simulink model "atrias_3d"  (R2014b)
settings: Solver=ode45  StartTime=0.0  StopTime=t_end  FixedStep=0.001  MaxStep=1e-2  RelTol=1e-3
InitFcn:
  | colors
  | simulation_params
  | mechanical_params
StartFcn:
  | tic
StopFcn:
  | stopscript
values from neighbouring files (symbols this model uses):
  b_hmotor = 0    [mechanical_params.m]
  b_leg_spring = 0.075*sqrt(k_leg_spring*0.5*.25^2)    [mechanical_params.m]
  b_rotor = 0*60/(2*pi)*9.725e-5    (= 0)    [mechanical_params.m]
  breakaway_friction = [25 25 25 25]    [mechanical_params.m]
  coulomb_friction = [20 20 20 20]    [mechanical_params.m]
  d_com = (d_hip_com_to_torso_com*m_torso)/(m_torso + num_legs*m_hshaft)    [mechanical_params.m]
  delta_phi_max = 160*pi/180    (= 2.79252680319)    [mechanical_params.m]
  delta_phi_min = 25.5*pi/180    (= 0.445058959259)    [mechanical_params.m]
  friction_linear_zone = [0.5 0.5 0.5 0.5].*pi/180    [mechanical_params.m]
  g = 9.81    [mechanical_params.m]
  HIP_MTR_MAX_TORQUE = max_current_hip*Kt_hip*N_h    (= 629.28)    [mechanical_params.m]
  initial_dx = -1    [mechanical_params.m]
  initial_hip_roll = 0    [mechanical_params.m]
  initial_pitch_joint_height = initial_com_height + boom_mount_to_com    [mechanical_params.m]
  initial_torso_pitch = 0*pi/180    (= 0)    [mechanical_params.m]
  initial_torso_roll = 0*pi/180    (= 0)    [mechanical_params.m]
  initial_torso_yaw = 0*pi/180    (= 0)    [mechanical_params.m]
  k_gx = m_total*g/0.01    (= 57082.15332)    [mechanical_params.m]
  k_gy = m_total*g/0.005    (= 114164.30664)    [mechanical_params.m]
  k_leg_spring = 2950    [mechanical_params.m]
  k_phi = 5000    [mechanical_params.m]
  Kb_leg = 0.121    [mechanical_params.m]
  Kt_leg = 0.121    [mechanical_params.m]
  L_leg = 0.102e-3    (= 0.000102)    [mechanical_params.m]
  l_seg = 0.5    [mechanical_params.m]
  LEG_MTR_MAX_TORQUE = max_current_leg * Kt_leg * N    (= 1210)    [mechanical_params.m]
  lowerleg_12 = 0.40    (= 0.4)    [mechanical_params.m]
  m_fblink = 0.46    [mechanical_params.m]
  m_hshaft = 18    [mechanical_params.m]
  m_lowerleg = 0.4438    [mechanical_params.m]
  m_output_gear = 1e-5    (= 1e-05)    [mechanical_params.m]
  m_rotor = 1e-5    (= 1e-05)    [mechanical_params.m]
  m_shin = 0.75    [mechanical_params.m]
  m_thigh = 0.69    [mechanical_params.m]
  m_torso = 17.5    [mechanical_params.m]
  m_total = num_legs*(m_hshaft + m_thigh + m_lowerleg + m_shin + m_fblink + 2*m_gearing) + m_torso    (= 58.18772)    [mechanical_params.m]
  m_virtual_gear = 1e-5    (= 1e-05)    [mechanical_params.m]
  max_current_leg = 200    [mechanical_params.m]
  max_voltage_leg = 50    [mechanical_params.m]
  mu_hmotor = 0.90    (= 0.9)    [mechanical_params.m]
  mu_motor = 0.85    [mechanical_params.m]
  mu_slide = 0.95    [mechanical_params.m]
  mu_stick = 1.00    (= 1)    [mechanical_params.m]
  N = 50    [mechanical_params.m]
  N_h = r_hip_shaft / r_hip_gearhead    (= 57)    [mechanical_params.m]
  phi_max_collision = -5*pi/180    (= -0.0872664625997)    [mechanical_params.m]
  phi_roll_max = pi + 16*pi/180    (= 3.42084533391)    [mechanical_params.m]
  phi_roll_min = pi - 9*pi/180    (= 2.98451302091)    [mechanical_params.m]
  phi_shin_max = 3*pi/2 + 17.5*pi/180    (= 5.01782159948)    [mechanical_params.m]
  phi_shin_min = pi - 45*pi/180    (= 2.35619449019)    [mechanical_params.m]
  phi_thigh_max = pi + 45*pi/180    (= 3.92699081699)    [mechanical_params.m]
  phi_thigh_min = pi/2 - 17.5*pi/180    (= 1.2653637077)    [mechanical_params.m]
  r_hip_gearhead = 0.009525    [mechanical_params.m]
  r_hip_shaft = 0.542925    [mechanical_params.m]
  R_leg = 0.052    [mechanical_params.m]
  r_rotor = 0.001    [mechanical_params.m]
  r_virtual_gear = N*r_rotor    (= 0.05)    [mechanical_params.m]
  shin_12 = 0.40    (= 0.4)    [mechanical_params.m]
  shin_initial_l = initial_l_leg_angle + acos(initial_l_leg_length)    [mechanical_params.m]
  shin_initial_r = initial_r_leg_angle + acos(initial_r_leg_length)    [mechanical_params.m]
  thigh_initial_l = initial_l_leg_angle - acos(initial_l_leg_length)    [mechanical_params.m]
  thigh_initial_r = initial_r_leg_angle - acos(initial_r_leg_length)    [mechanical_params.m]
  v_gx_max = 0.03    [mechanical_params.m]
  v_gy_max = 0.03    [mechanical_params.m]
  v_phi_max = 1/60    (= 0.0166666666667)    [mechanical_params.m]
  viscous_friction = [0.001 0.001 0.001 0.001]    [mechanical_params.m]
  vLimit = 0.01    [mechanical_params.m]
undefined symbols (not defined in the file or in its folder): A_lpf_velocity, B1_lpf_velocity, B2_lpf_velocity, fblink_color_d, floor_color_d, hshaft_color_d, lowerleg_color_d, output_sample_time, rad, s, sample_time, sgn, shin_color_d, t_friction, thigh_color_d, torso_color_d, X, Y, Z
libraries: sm_lib x163, nesl_utility x116, simulink x47, fl_lib x16, simulink_extras x2, mblibv1 x2, commnoisgen2 x1
(part 1 of 7)
settings Model: Creator=wmartin  LastModifiedBy=jonesmik
settings SolverCC: InitialStep=sample_time  MaxOrder=2  ConsecutiveZCsStepRelTol=auto  MaxConsecutiveZCs=auto  ZeroCrossControl=DisableAll  ZeroCrossAlgorithm=Adaptive  InsertRTBMode=Never (minimum delay)
settings DataIOCC: LimitDataPoints=off  SaveOutput=off  SignalLogging=off  DSMLogging=off  OutputOption=SpecifiedOutputTimes  OutputTimes=[0:output_sample_time:t_end]
settings OptimizationCC: InlineParams=on  UseDivisionForNetSlopeComputation=UseDivisionForReciprocalsOfIntegersOnly  UseFloatMulNetSlope=on  InlineInvariantSignals=on  EnhancedBackFolding=on  MemcpyThreshold=1024  StateBitsets=on  DataBitsets=on  EfficientFloat2IntCast=on  SimCompilerOptimization=On  AccelVerboseBuild=on
settings DebuggingCC: AlgebraicLoopMsg=none  UnderspecifiedInitializationDetection=Classic  MergeDetectMultiDrivingBlocksExec=none  SolverPrmCheckMsg=none  UnconnectedInputMsg=none  UnconnectedOutputMsg=none  UnconnectedLineMsg=none  StateNameClashWarn=warning
settings SFSimCC: SFSimEnableDebug=off  SFSimOverflowDetection=off  SFSimEcho=off
settings RTWCC: BuildConfiguration=Faster Runs
settings SimscapeCC: EditingMode=Restricted
settings ExplorerConfigSet: InternalSimMechanicsExplorerSettings="<ExplorerConfiguration><canonicalview>default</canonicalview><AnimationSetting><BasePlaybackSpeed>1.0</BasePlaybackSpeed><PlaybackSpeedFactor>1.0</PlaybackSpeedFactor></AnimationSetting><TilePanel><TileInfo><Tiles Columns=\"1\" Count=\"1\" Rows=\"1\"><Column Left=\"2\" Weight=\"1\"/><Column Left=\"876\"/><Row Top=\"2\" Weight=\"1\"/><Row Top=\"1114\"/><Tile Height=\"1\" Width=\"1\" X=\"0\" Y=\"0\"/></Tiles></TileInfo><SceneInfo><SceneViewer><BGColor><R>0.89803922176361084</R><G>0.89803922176361084</G><B>0.94901961088180542</B></BGColor><Camera><Position><X>-30.49227767907372</X><Y>0.073515473804125403</Y><Z>1.0865448159450428</Z></Position><Center><X>0</X><Y>0.073515473804125403</Y><Z>1.0865448159450428</Z></Center><Up><X>0</X><Y>0</Y><Z>1</Z></Up><Left>-3.5820650684649178</Left><Right>3.5820650684649178</Right><Bottom>-0.28042415136526933</Bottom><Top>0.28042415136526933</Top></Camera></SceneViewer></SceneInfo></TilePanel></ExplorerConfiguration>"

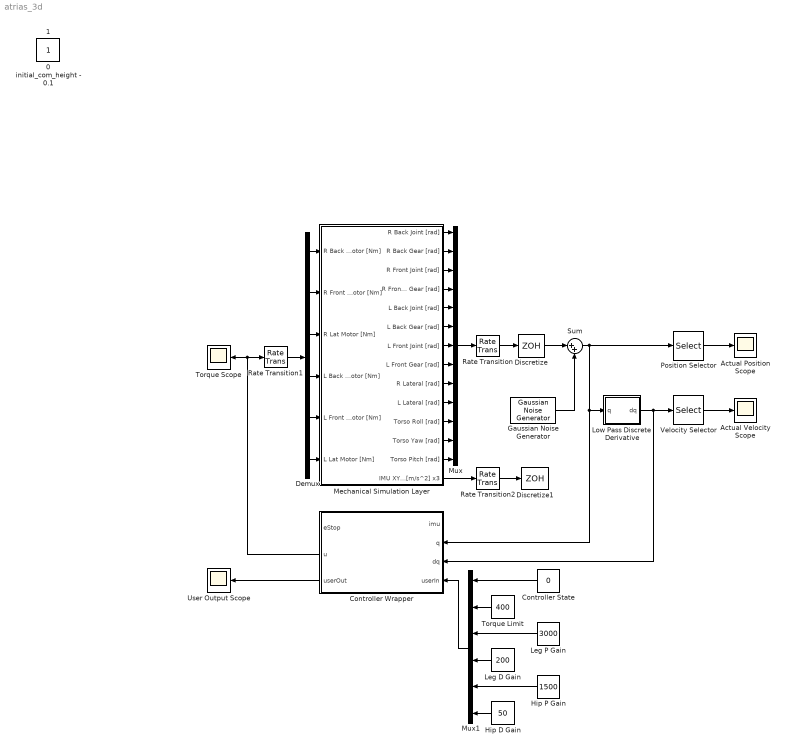
== system atrias_3d ==
  Actual Position Scope : Scope
      settings: SaveName=ScopeData7
  Actual Velocity Scope : Scope
      settings: YMin=-8  YMax=4  SaveName=ScopeData8
  Controller State : Constant  Value=0
  Controller Wrapper : MATLAB Function  TreatAsAtomicUnit=on
  Demux : Demux  Outputs=6
  Discretize : ZeroOrderHold  SampleTime=sample_time
  Discretize1 : ZeroOrderHold  SampleTime=sample_time
  Gaussian Noise Generator : commnoisgen2/Gaussian Noise Generator  m=0  d=sensor_noise_variance  s=41  Ts=sample_time  frameBased=off  sampPerFrame=1  orient=off  outDataType=double
  Hip D Gain : Constant  Value=50
  Hip P Gain : Constant  Value=1500
  Leg D Gain : Constant  Value=200
  Leg P Gain : Constant  Value=3000
  Low Pass Discrete Derivative : Subsystem
  Mechanical Simulation Layer : Subsystem
      mask Display: image('biped.jpg')
  Mux : Mux  Inputs=13
  Mux1 : Mux  Inputs=6
  Position Selector : Selector  InputPortWidth=13  IndexOptions=Select all  Indices=[13]
  Rate Transition : RateTransition  OutPortSampleTime=sample_time
  Rate Transition1 : RateTransition  OutPortSampleTime=sample_time
  Rate Transition2 : RateTransition  OutPortSampleTime=sample_time
  Sum : Sum  Inputs=|++
  Torque Scope : Scope
      settings: SaveName=ScopeData5
  Torque Limit : Constant  Value=400
  User Output Scope : Scope
      settings: YMin=0.12  YMax=0.28  SaveName=ScopeData4
  Velocity Selector : Selector  InputPortWidth=13  IndexOptions=Select all  Indices=[13]
  0 : Constant  IOType=siggen
  1 : Constant  IOType=siggen
  initial_com_height - 0.1 : Constant  IOType=siggen
  wires:
  Mechanical Simulation Layer/1(R Back Joint [rad]) -> Mux/1
  Mechanical Simulation Layer/2(R Back Gear [rad]) -> Mux/2
  Mechanical Simulation Layer/3(R Front Joint [rad]) -> Mux/3
  Mechanical Simulation Layer/4(R Front Gear [rad]) -> Mux/4
  Mechanical Simulation Layer/5(L Back Joint [rad]) -> Mux/5
  Mechanical Simulation Layer/6(L Back Gear [rad]) -> Mux/6
  Mechanical Simulation Layer/7(L Front Joint [rad]) -> Mux/7
  Mechanical Simulation Layer/8(L Front Gear [rad]) -> Mux/8
  Mechanical Simulation Layer/9(R Lateral [rad]) -> Mux/9
  Mechanical Simulation Layer/10(L Lateral [rad]) -> Mux/10
  Mechanical Simulation Layer/11(Torso Roll [rad]) -> Mux/11
  Mechanical Simulation Layer/12(Torso Yaw [rad]) -> Mux/12
  Mechanical Simulation Layer/13(Torso Pitch [rad]) -> Mux/13
  Demux/1 -> Mechanical Simulation Layer/1(R Back Motor [Nm])
  Demux/2 -> Mechanical Simulation Layer/2(R Front Motor [Nm])
  Demux/3 -> Mechanical Simulation Layer/3(R Lat Motor [Nm])
  Demux/4 -> Mechanical Simulation Layer/4(L Back Motor [Nm])
  Demux/5 -> Mechanical Simulation Layer/5(L Front Motor [Nm])
  Demux/6 -> Mechanical Simulation Layer/6(L Lat Motor [Nm])
  Rate Transition1/1 -> Demux/1
  Discretize/1 -> Sum/1
  Gaussian Noise Generator/1 -> Sum/2
  Rate Transition/1 -> Discretize/1
  Mux/1 -> Rate Transition/1
  Mechanical Simulation Layer/14("IMU XYZ Acclerations [m/s^2] x3 ") -> Rate Transition2/1
  Rate Transition2/1 -> Discretize1/1
  Sum/1 -> Position Selector/1, Controller Wrapper/2(q), Low Pass Discrete Derivative/1(q)
  Low Pass Discrete Derivative/1(dq) -> Velocity Selector/1, Controller Wrapper/3(dq)
  Controller Wrapper/2(u) -> Rate Transition1/1, Torque Scope/1
  Controller Wrapper/3(userOut) -> User Output Scope/1
  Mux1/1 -> Controller Wrapper/4(userIn)
  Controller State/1 -> Mux1/1
  Torque Limit/1 -> Mux1/2
  Leg P Gain/1 -> Mux1/3
  Leg D Gain/1 -> Mux1/4
  Hip P Gain/1 -> Mux1/5
  Hip D Gain/1 -> Mux1/6
  Position Selector/1 -> Actual Position Scope/1
  Velocity Selector/1 -> Actual Velocity Scope/1

== system atrias_3d/Low Pass Discrete Derivative ==
  q : Inport
  Gain1 : Gain  Gain=1/sample_time
  discrete difference : Subsystem
  two_pole_filter : DiscreteTransferFcn  Numerator=[A_lpf_velocity 0 0]  Denominator=[1 B1_lpf_velocity B2_lpf_velocity]  SampleTime=sample_time
  dq : Outport
  wires:
  discrete difference/1(out) -> Gain1/1
  Gain1/1 -> two_pole_filter/1
  two_pole_filter/1 -> dq/1
  q/1 -> discrete difference/1(in)

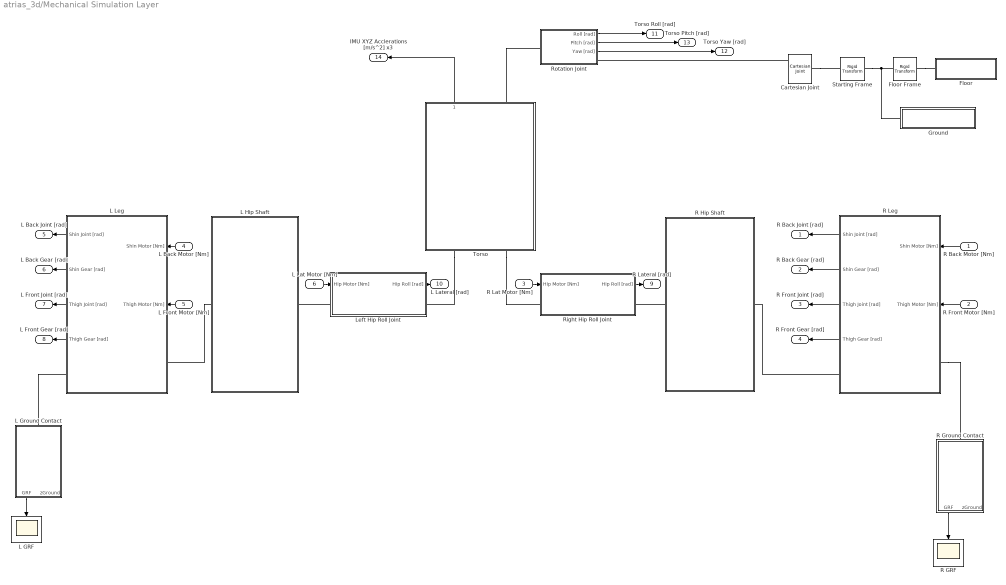
== system atrias_3d/Mechanical Simulation Layer ==
  R Back Motor [Nm] : Inport
  R Front Motor [Nm] : Inport  Port=2
  R Lat Motor [Nm] : Inport  Port=3
  L Back Motor [Nm] : Inport  Port=4
  L Front Motor [Nm] : Inport  Port=5
  L Lat Motor [Nm] : Inport  Port=6
  Cartesian Joint : sm_lib/Joints/Cartesian Joint  SenseConstraintForce=off  SenseConstraintForceX=off  SenseConstraintForceY=off  SenseConstraintForceZ=off  SenseConstraintTorque=off  SenseConstraintTorqueX=off  SenseConstraintTorqueY=off  SenseConstraintTorqueZ=off  SenseTotalForce=off  SenseTotalForceX=off  SenseTotalForceY=off  SenseTotalForceZ=off  SenseTotalTorque=off  SenseTotalTorqueX=off  SenseTotalTorqueY=off  SenseTotalTorqueZ=off  CompositeWrenchDir=FollowerOnBase  CompositeWrenchFrame=BaseFrame  PxEquilibriumPosition=0  PxEquilibriumPositionUnits=m  PxSpringStiffness=0  PxSpringStiffnessUnits=N/m  PxDampingCoefficient=0  PxDampingCoefficientUnits=N/(m/s)  PxTorqueActuationMode=NoTorque  PxMotionActuationMode=ComputedMotion  PxSensePosition=off  PxSenseVelocity=on  PxSenseAcceleration=off  PxSenseTorqueForce=off  PxPositionTargetValue=0  PxPositionTargetValueUnits=m  PxPositionTargetSpecify=off  PxPositionTargetPriority=High  PxVelocityTargetValue=initial_dx  PxVelocityTargetValueUnits=m/s  PxVelocityTargetSpecify=on  PxVelocityTargetPriority=High  PyEquilibriumPosition=0  PyEquilibriumPositionUnits=m  PySpringStiffness=0  PySpringStiffnessUnits=N/m  PyDampingCoefficient=0  PyDampingCoefficientUnits=N/(m/s)  PyTorqueActuationMode=NoTorque  PyMotionActuationMode=ComputedMotion  PySensePosition=off  PySenseVelocity=off  PySenseAcceleration=off  PySenseTorqueForce=off  PyPositionTargetValue=0  PyPositionTargetValueUnits=m  PyPositionTargetSpecify=off  PyPositionTargetPriority=High  PyVelocityTargetValue=0  PyVelocityTargetValueUnits=m/s  PyVelocityTargetSpecify=off  PyVelocityTargetPriority=High  PzEquilibriumPosition=0  PzEquilibriumPositionUnits=m  PzSpringStiffness=0  PzSpringStiffnessUnits=N/m  PzDampingCoefficient=0  PzDampingCoefficientUnits=N/(m/s)  PzTorqueActuationMode=NoTorque  PzMotionActuationMode=ComputedMotion  PzSensePosition=off  PzSenseVelocity=on  PzSenseAcceleration=off  PzSenseTorqueForce=off  PzPositionTargetValue=0  PzPositionTargetValueUnits=m  PzPositionTargetSpecify=off  PzPositionTargetPriority=High  PzVelocityTargetValue=-initial_dx  PzVelocityTargetValueUnits=m/s  PzVelocityTargetSpecify=off  PzVelocityTargetPriority=High  BlockFunction=simmechanics.library.joints.cartesian_joint
  Floor : Subsystem
  Floor Frame : sm_lib/Frames and Transforms/Rigid Transform  TranslationMethod=Cartesian  TranslationLengthUnit=m  TranslationStandardAxis=+Z  TranslationStandardOffset=0  TranslationCartesianOffset=[0 0 -0.015]  TranslationROffset=0  TranslationROffsetUnits=m  TranslationZOffset=0  TranslationZOffsetUnits=m  TranslationThetaOffset=0  TranslationThetaOffsetUnits=deg  RotationMethod=None  RotationAngleUnits=deg  RotationStandardAxis=+Z  RotationAngle=0  RotationArbitraryAxis=[0 0 1]  FollAlignAxisA=+Z  BaseAlignAxisA=+Y  FollAlignAxisB=+X  BaseAlignAxisB=+X  RotationMatrix=[1 0 0; 0 1 0; 0 0 1]  BlockFunction=simmechanics.library.frames_transforms.rigid_transform
  Ground : Subsystem
  L GRF : Scope
      settings: YMin=-175  YMax=350
  L Ground Contact : Subsystem  SystemSampleTime=t_friction
  L Hip Shaft : Subsystem
      mask Display: image(flipdim(imread('hip_shaft.jpg'),2));
  L Leg : Subsystem
      mask Display: image('leg.jpg');
  Left Hip Roll Joint : Subsystem
  R GRF : Scope
      settings: TimeRange=2.5  YMin=-4000  YMax=5000
  R Ground Contact : Subsystem  SystemSampleTime=t_friction
  R Hip Shaft : Subsystem
      mask Display: image('hip_shaft.jpg');
  R Leg : Subsystem
      mask Display: image('leg.jpg');
  Right Hip Roll Joint : Subsystem
  Rotation Joint : Subsystem
  Starting Frame : sm_lib/Frames and Transforms/Rigid Transform  TranslationMethod=Cartesian  TranslationLengthUnit=m  TranslationStandardAxis=+Z  TranslationStandardOffset=0  TranslationCartesianOffset=[0 0 initial_pitch_joint_height]  TranslationROffset=0  TranslationROffsetUnits=m  TranslationZOffset=0  TranslationZOffsetUnits=m  TranslationThetaOffset=0  TranslationThetaOffsetUnits=deg  RotationMethod=None  RotationAngleUnits=deg  RotationStandardAxis=+Z  RotationAngle=0  RotationArbitraryAxis=[0 0 1]  FollAlignAxisA=+Z  BaseAlignAxisA=+Y  FollAlignAxisB=+X  BaseAlignAxisB=+X  RotationMatrix=[1 0 0; 0 1 0; 0 0 1]  BlockFunction=simmechanics.library.frames_transforms.rigid_transform
  Torso : Subsystem
      mask Display: image('torso.png');
  R Back Joint [rad] : Outport
  R Back Gear [rad] : Outport  Port=2
  R Front Joint [rad] : Outport  Port=3
  R Front Gear [rad] : Outport  Port=4
  L Back Joint [rad] : Outport  Port=5
  L Back Gear [rad] : Outport  Port=6
  L Front Joint [rad] : Outport  Port=7
  L Front Gear [rad] : Outport  Port=8
  R Lateral [rad] : Outport  Port=9
  L Lateral [rad] : Outport  Port=10
  Torso Roll [rad] : Outport  Port=11
  Torso Yaw [rad] : Outport  Port=12
  Torso Pitch [rad] : Outport  Port=13
  "IMU XYZ Acclerations [m/s^2] x3 " : Outport  Port=14
  wires:
  L Leg/1(Shin Joint [rad]) -> L Back Joint [rad]/1
  R Back Motor [Nm]/1 -> R Leg/1(Shin Motor [Nm])
  L Back Motor [Nm]/1 -> L Leg/1(Shin Motor [Nm])
  Right Hip Roll Joint/1(Hip Roll [rad]) -> R Lateral [rad]/1
  L Leg/3(Thigh Joint [rad]) -> L Front Joint [rad]/1
  Left Hip Roll Joint/1(Hip Roll [rad]) -> L Lateral [rad]/1
  L Leg/4(Thigh Gear [rad]) -> L Front Gear [rad]/1
  R Leg/1(Shin Joint [rad]) -> R Back Joint [rad]/1
  R Leg/2(Shin Gear [rad]) -> R Back Gear [rad]/1
  L Leg/2(Shin Gear [rad]) -> L Back Gear [rad]/1
  R Leg/4(Thigh Gear [rad]) -> R Front Gear [rad]/1
  L Front Motor [Nm]/1 -> L Leg/2("Thigh Motor [Nm]  ")
  R Lat Motor [Nm]/1 -> Right Hip Roll Joint/1(Hip Motor [Nm])
  R Front Motor [Nm]/1 -> R Leg/2("Thigh Motor [Nm]  ")
  L Lat Motor [Nm]/1 -> Left Hip Roll Joint/1(Hip Motor [Nm])
  R Ground Contact/1(GRF) -> R GRF/1
  L Ground Contact/1(GRF) -> L GRF/1
  R Leg/3(Thigh Joint [rad]) -> R Front Joint [rad]/1
  Rotation Joint/2(Pitch [rad]) -> Torso Pitch [rad]/1
  Rotation Joint/1(Roll [rad]) -> Torso Roll [rad]/1
  Rotation Joint/3(Yaw [rad]) -> Torso Yaw [rad]/1
  Torso/1(IMU XYZ Accelerations [m/s^2] x3) -> "IMU XYZ Acclerations [m/s^2] x3 "/1
  connections:
  Torso/LConn1 -- Left Hip Roll Joint/RConn1
  R Hip Shaft/RConn1 -- Right Hip Roll Joint/RConn1
  Left Hip Roll Joint/LConn1 -- L Hip Shaft/LConn1
  R Leg/LConn1 -- R Ground Contact/LConn1
  R Leg/RConn1 -- R Hip Shaft/LConn1
  Torso/LConn2 -- Right Hip Roll Joint/LConn1
  L Hip Shaft/RConn1 -- L Leg/LConn1
  L Leg/RConn1 -- L Ground Contact/LConn1
  Rotation Joint/LConn1 -- Torso/RConn1
  Floor Frame/RConn1 -- Floor/LConn1
  Floor Frame/LConn1 -- Starting Frame/LConn1 -- Ground/RConn1
  Cartesian Joint/RConn1 -- Rotation Joint/RConn1
  Cartesian Joint/LConn1 -- Starting Frame/RConn1

== system atrias_3d/Low Pass Discrete Derivative/discrete difference ==
  note: q Order:
      |
      | backJointR
      | backGearR
      | frontJointR
      | frontGearR
      |
      | backJointL
      | backGearL
      | frontJointL
      | frontGearL
      |
      | latR
      | latL
      |
      | boomRoll
      | boomYaw
      | boomPitch
  in : Inport
  Demux : Demux  Outputs=13
  Mux : Mux  Inputs=13
  difference : simulink/Discrete/Difference  ICPrevInput=shin_initial_r  InputProcessing=Columns as channels (frame based)  OutMin=[]  OutMax=[]  OutDataType=fixdt(1, 16)  OutScaling=2^-10  DoSatur=off
  difference1 : simulink/Discrete/Difference  ICPrevInput=shin_initial_r  InputProcessing=Columns as channels (frame based)  OutMin=[]  OutMax=[]  OutDataType=fixdt(1, 16)  OutScaling=2^-10  DoSatur=off
  difference10 : simulink/Discrete/Difference  ICPrevInput=initial_torso_roll  InputProcessing=Columns as channels (frame based)  OutMin=[]  OutMax=[]  OutDataType=fixdt(1, 16)  OutScaling=2^-10  DoSatur=off
  difference11 : simulink/Discrete/Difference  ICPrevInput=initial_torso_yaw  InputProcessing=Columns as channels (frame based)  OutMin=[]  OutMax=[]  OutDataType=fixdt(1, 16)  OutScaling=2^-10  DoSatur=off
  difference12 : simulink/Discrete/Difference  ICPrevInput=initial_torso_pitch  InputProcessing=Columns as channels (frame based)  OutMin=[]  OutMax=[]  OutDataType=fixdt(1, 16)  OutScaling=2^-10  DoSatur=off
  difference2 : simulink/Discrete/Difference  ICPrevInput=thigh_initial_r  InputProcessing=Columns as channels (frame based)  OutMin=[]  OutMax=[]  OutDataType=fixdt(1, 16)  OutScaling=2^-10  DoSatur=off
  difference3 : simulink/Discrete/Difference  ICPrevInput=thigh_initial_r  InputProcessing=Columns as channels (frame based)  OutMin=[]  OutMax=[]  OutDataType=fixdt(1, 16)  OutScaling=2^-10  DoSatur=off
  difference4 : simulink/Discrete/Difference  ICPrevInput=shin_initial_l  InputProcessing=Columns as channels (frame based)  OutMin=[]  OutMax=[]  OutDataType=fixdt(1, 16)  OutScaling=2^-10  DoSatur=off
  difference5 : simulink/Discrete/Difference  ICPrevInput=shin_initial_l  InputProcessing=Columns as channels (frame based)  OutMin=[]  OutMax=[]  OutDataType=fixdt(1, 16)  OutScaling=2^-10  DoSatur=off
  difference6 : simulink/Discrete/Difference  ICPrevInput=thigh_initial_l  InputProcessing=Columns as channels (frame based)  OutMin=[]  OutMax=[]  OutDataType=fixdt(1, 16)  OutScaling=2^-10  DoSatur=off
  difference7 : simulink/Discrete/Difference  ICPrevInput=thigh_initial_l  InputProcessing=Columns as channels (frame based)  OutMin=[]  OutMax=[]  OutDataType=fixdt(1, 16)  OutScaling=2^-10  DoSatur=off
  difference8 : simulink/Discrete/Difference  ICPrevInput=initial_hip_roll  InputProcessing=Columns as channels (frame based)  OutMin=[]  OutMax=[]  OutDataType=fixdt(1, 16)  OutScaling=2^-10  DoSatur=off
  difference9 : simulink/Discrete/Difference  ICPrevInput=initial_hip_roll  InputProcessing=Columns as channels (frame based)  OutMin=[]  OutMax=[]  OutDataType=fixdt(1, 16)  OutScaling=2^-10  DoSatur=off
  out : Outport
  wires:
  difference/1 -> Mux/1
  difference12/1 -> Mux/13
  Demux/13 -> difference12/1
  difference11/1 -> Mux/12
  Demux/12 -> difference11/1
  difference10/1 -> Mux/11
  Demux/11 -> difference10/1
  difference9/1 -> Mux/10
  Demux/10 -> difference9/1
  difference8/1 -> Mux/9
  Demux/9 -> difference8/1
  difference7/1 -> Mux/8
  Demux/8 -> difference7/1
  difference6/1 -> Mux/7
  Demux/7 -> difference6/1
  difference5/1 -> Mux/6
  Demux/6 -> difference5/1
  difference4/1 -> Mux/5
  Demux/5 -> difference4/1
  difference3/1 -> Mux/4
  Demux/4 -> difference3/1
  difference2/1 -> Mux/3
  Demux/3 -> difference2/1
  difference1/1 -> Mux/2
  Demux/2 -> difference1/1
  Mux/1 -> out/1
  in/1 -> Demux/1
  Demux/1 -> difference/1

== system atrias_3d/Mechanical Simulation Layer/Floor ==
  Floor Tile 1 : sm_lib/Body Elements/Solid  InertiaType=PointMass  Mass=0  MassUnits=kg  CenterOfMass=[0 0 0]  CenterOfMassUnits=m  MomentsOfInertia=[0 0 0]  MomentsOfInertiaUnits=kg*m^2  ProductsOfInertia=[0 0 0]  ProductsOfInertiaUnits=kg*m^2  DensityBased=on  Density=1000  DensityUnits=kg/(m^3)  GraphicType=FromGeometry  MarkerShape=Sphere  MarkerSize=10  MarkerSizeUnits=m  GraphicVisPropType=AdvancedVisualProperties  GraphicDiffuseColor=floor_color_d  GraphicSpecularColor=[0.5 0.5 0.5 1.0]  GraphicAmbientColor=[floor_color_d*0.5 1.0]  GraphicEmissiveColor=[0.0 0.0 0.0 1.0]  GraphicShininess=128  GraphicOpacity=1.0  GeometryShape=Brick  RectangleSize=[1 1]  RectangleSizeUnits=m  BrickDimensions=[20 20 0.03]  BrickDimensionUnits=m  CylinderRadius=3.5  CylinderRadiusUnits=m  CylinderLength=0.03  CylinderLengthUnits=m  SphereRadius=1  SphereRadiusUnits=m  EllipsoidRadii=[1 1 1]  EllipsoidRadiiUnits=m  ExtrusionCrossSection=[1 1; -1 1; -1 -1; 1 -1]  ExtrusionCrossSectionUnits=m  ExtrusionLength=1  ExtrusionLengthUnits=m  PolygonNumSides=3  PolygonOuterRadius=1  PolygonOuterRadiusUnits=m  ExtGeomFileType=STL  ExtGeomFileUnits=m  RevolutionCrossSection=0  RevolutionCrossSectionUnits=m  RevolutionExtent=Custom  RevolutionAngle=0  RevolutionAngleUnits=rad  BlockFunction=simmechanics.library.body_elements.solid
  Floor Bottom : PMIOPort  Port=1  Side=Left
  connections:
  Floor Tile 1/RConn1 -- Floor Bottom/RConn1

== system atrias_3d/Mechanical Simulation Layer/Ground ==
  Mechanism Configuration : sm_lib/Utilities/Mechanism Configuration  UniformGravity=Constant  GravityVector=[0 0 -g]  GravityUnits=m/s^2  LinearizationDelta=0.001  BlockFunction=simmechanics.library.utilities.mechanism_configuration
  Solver Configuration : nesl_utility/Solver Configuration  PhysicalDomain=network_engine_domain  SubClassName=solver  LeftPortType=input  RightPortType=generic  Accelerate=off  Tones=[]  Harmonics=[]  SimulateNoise=off  Profile=off  UseLocalSampling=off  EnableSwitchedLinearOptims=on  FrequencyDomain=off  UseCCode=off  RelTol=0.001  AbsTol=1e-06  MinStep=1e-09  ToWorkspace=off  DoDC=on  ResidualTolerance=1e-09  UseLocalSolver=off  LocalSolverChoice=NE_TRAPEZOIDAL_ADVANCER  LocalSolverSampleTime=0.001  DoFixedCost=off  MaxNonlinIter=3  MaxModeIter=2  LinearAlgebra=Sparse  DelaysMemoryBudget=1024  AutomaticFiltering=on  FilteringTimeConstant=0.001
  World Frame : sm_lib/Frames and Transforms/World Frame  BlockFunction=simmechanics.library.frames_transforms.world_frame
  Ground Connection : PMIOPort  Port=1  Side=Right
  connections:
  World Frame/RConn1 -- Ground Connection/RConn1 -- Solver Configuration/RConn1 -- Mechanism Configuration/RConn1

== system atrias_3d/Mechanical Simulation Layer/L Ground Contact ==
  note: Ground Interaction Model
  External Force and Torque : sm_lib/Forces and Torques/External Force and Torque  ForceResolutionFrame=World  EnableForceX=off  EnableForceY=off  EnableForceZ=off  EnableForce=on  TorqueResolutionFrame=AttachedFrame  EnableTorqueX=off  EnableTorqueY=off  EnableTorqueZ=off  EnableTorque=off  BlockFunction=simmechanics.library.forces_torques.external_force_torque
  Ground Friction Model : Subsystem
  Mux1 : Mux  Inputs=3
  PS-Simulink Converter{,1..5} (6 alike) : nesl_utility/PS-Simulink Converter  PhysicalDomain=network_engine_domain  SubClassName=ps_output  LeftPortType=input  RightPortType=output  PseudoPeriodic=off  Frequencies=[]  Unit=1  AffineConversion=off
  Simulink-PS Converter : nesl_utility/Simulink-PS Converter  PhysicalDomain=network_engine_domain  SubClassName=ps_input  LeftPortType=input  RightPortType=output  PseudoPeriodic=off  Frequencies=[]  NoiseDistribution=none  NoiseParameters=[]  Unit=1  AffineConversion=off  InputFiltering=off  SimscapeFilterOrder=1  InputFilterTimeConstant=0.001  UdotUserProvided=1
  Stiction : Scope
      settings: TimeRange=2.5  YMin=0  YMax=130  SaveName=ScopeData15
  Sum : Sum  Inputs=-+|
  Terminator : Terminator
  Transform Sensor : sm_lib/Frames and Transforms/Transform Sensor  MeasurementFrame=World  SenseAngle=off  SenseAxis=off  SenseAngle1=off  SenseAngle2=off  SenseAngle3=off  SenseQ=off  SenseR=off  SenseOmegaX=off  SenseOmegaY=off  SenseOmegaZ=off  SenseOmega1=off  SenseOmega2=off  SenseOmega3=off  SenseQDot=off  SenseRDot=off  SenseAlphaX=off  SenseAlphaY=off  SenseAlphaZ=off  SenseAlpha1=off  SenseAlpha2=off  SenseAlpha3=off  SenseQDDot=off  SenseRDDot=off  SenseX=on  SenseY=on  SenseZ=on  SenseRad=off  SenseAzim=off  SenseDist=off  SenseInc=off  SenseXDot=on  SenseYDot=on  SenseZDot=on  SenseRadDot=off  SenseAzimDot=off  SenseDistDot=off  SenseIncDot=off  SenseXDDot=off  SenseYDDot=off  SenseZDDot=off  SenseRadDDot=off  SenseAzimDDot=off  SenseDistDDot=off  SenseIncDDot=off  BlockFunction=simmechanics.library.frames_transforms.transform_sensor
  World Frame : sm_lib/Frames and Transforms/World Frame  BlockFunction=simmechanics.library.frames_transforms.world_frame
  groundHeight : Constant  Value=0
  skin contact sensor : simulink/Logic and Bit Operations/Compare To Zero  relop=<=  OutDataTypeStr=boolean
  Foot Point : PMIOPort  Port=1  Side=Left
  GRF : Outport
  zGround : Outport  Port=2
  tag scope: GRFz_L=global
  wires:
  Ground Friction Model/3(Fn_Ground[N]) -> Mux1/3, [GRFz_L]
  Ground Friction Model/2(FyFriction [N]) -> Mux1/2
  PS-Simulink Converter5/1 -> Ground Friction Model/6(vy [m/s])
  skin contact sensor/1 -> Ground Friction Model/Enable
  Mux1/1 -> GRF/1, Simulink-PS Converter/1
  groundHeight/1 -> Sum/1, zGround/1
  PS-Simulink Converter4/1 -> Ground Friction Model/2(vnormal [m/s])
  PS-Simulink Converter3/1 -> Ground Friction Model/4(vx [m/s])
  PS-Simulink Converter2/1 -> Ground Friction Model/3(x [m])
  PS-Simulink Converter1/1 -> Ground Friction Model/5(y [m])
  PS-Simulink Converter/1 -> Sum/2
  Ground Friction Model/4(Stiction!) -> Terminator/1, Stiction/1
  Ground Friction Model/1(FxFriction [N]) -> Mux1/1
  Sum/1 -> Ground Friction Model/1(delta normal [m]), skin contact sensor/1
  connections:
  World Frame/RConn1 -- Transform Sensor/LConn1
  Transform Sensor/RConn7 -- PS-Simulink Converter4/LConn1
  Transform Sensor/RConn6 -- PS-Simulink Converter5/LConn1
  PS-Simulink Converter3/LConn1 -- Transform Sensor/RConn5
  PS-Simulink Converter2/LConn1 -- Transform Sensor/RConn2
  Transform Sensor/RConn4 -- PS-Simulink Converter/LConn1
  Transform Sensor/RConn3 -- PS-Simulink Converter1/LConn1
  External Force and Torque/LConn1 -- Simulink-PS Converter/RConn1
  Foot Point/RConn1 -- Transform Sensor/RConn1 -- External Force and Torque/RConn1

== system atrias_3d/Mechanical Simulation Layer/L Hip Shaft ==
  CS1 to CS2 : sm_lib/Frames and Transforms/Rigid Transform  TranslationMethod=Cartesian  TranslationLengthUnit=m  TranslationStandardAxis=+Z  TranslationStandardOffset=0  TranslationCartesianOffset=hshaft_12  TranslationROffset=0  TranslationROffsetUnits=m  TranslationZOffset=0  TranslationZOffsetUnits=m  TranslationThetaOffset=0  TranslationThetaOffsetUnits=deg  RotationMethod=None  RotationAngleUnits=deg  RotationStandardAxis=+Z  RotationAngle=0  RotationArbitraryAxis=[0 0 1]  FollAlignAxisA=+X  BaseAlignAxisA=+Y  FollAlignAxisB=+Y  BaseAlignAxisB=+Z  RotationMatrix=[1 0 0; 0 1 0; 0 0 1]  BlockFunction=simmechanics.library.frames_transforms.rigid_transform
  Frame Data : Subsystem
  Rotate 180 degrees : sm_lib/Frames and Transforms/Rigid Transform  TranslationMethod=None  TranslationLengthUnit=m  TranslationStandardAxis=+Z  TranslationStandardOffset=0  TranslationCartesianOffset=hshaft_12  TranslationROffset=0  TranslationROffsetUnits=m  TranslationZOffset=0  TranslationZOffsetUnits=m  TranslationThetaOffset=0  TranslationThetaOffsetUnits=deg  RotationMethod=StandardAxis  RotationAngleUnits=deg  RotationStandardAxis=+Y  RotationAngle=180  RotationArbitraryAxis=[0 0 1]  FollAlignAxisA=+X  BaseAlignAxisA=+Y  FollAlignAxisB=+Y  BaseAlignAxisB=+Z  RotationMatrix=[1 0 0; 0 1 0; 0 0 1]  BlockFunction=simmechanics.library.frames_transforms.rigid_transform
  Rotate back 180 degrees : sm_lib/Frames and Transforms/Rigid Transform  TranslationMethod=None  TranslationLengthUnit=m  TranslationStandardAxis=+Z  TranslationStandardOffset=0  TranslationCartesianOffset=hshaft_12  TranslationROffset=0  TranslationROffsetUnits=m  TranslationZOffset=0  TranslationZOffsetUnits=m  TranslationThetaOffset=0  TranslationThetaOffsetUnits=deg  RotationMethod=StandardAxis  RotationAngleUnits=deg  RotationStandardAxis=+Y  RotationAngle=180  RotationArbitraryAxis=[0 0 1]  FollAlignAxisA=+X  BaseAlignAxisA=+Y  FollAlignAxisB=+Y  BaseAlignAxisB=+Z  RotationMatrix=[1 0 0; 0 1 0; 0 0 1]  BlockFunction=simmechanics.library.frames_transforms.rigid_transform
  Solid : sm_lib/Body Elements/Solid  InertiaType=Custom  Mass=m_hshaft  MassUnits=kg  CenterOfMass=com_hshaft  CenterOfMassUnits=m  MomentsOfInertia=i_hshaft_moments  MomentsOfInertiaUnits=kg*m^2  ProductsOfInertia=i_hshaft_products  ProductsOfInertiaUnits=kg*m^2  DensityBased=on  Density=1000  DensityUnits=kg/(m^3)  GraphicType=FromGeometry  MarkerShape=Sphere  MarkerSize=10  MarkerSizeUnits=m  GraphicVisPropType=AdvancedVisualProperties  GraphicDiffuseColor=hshaft_color_d  GraphicSpecularColor=[[1 1 1]*0.5 1.0]  GraphicAmbientColor=[hshaft_color_d*0.50 1.0]  GraphicEmissiveColor=[0 0 0 1.0]  GraphicShininess=128  GraphicOpacity=1.0  GeometryShape=FromFile  RectangleSize=[1 1]  RectangleSizeUnits=m  BrickDimensions=[1 1 1]  BrickDimensionUnits=m  CylinderRadius=l_rad  CylinderRadiusUnits=m  CylinderLength=l_seg  CylinderLengthUnits=m  SphereRadius=1  SphereRadiusUnits=m  EllipsoidRadii=[1 1 1]  EllipsoidRadiiUnits=m  ExtrusionCrossSection=[1 1; -1 1; -1 -1; 1 -1]  ExtrusionCrossSectionUnits=m  ExtrusionLength=1  ExtrusionLengthUnits=m  PolygonNumSides=3  PolygonOuterRadius=1  PolygonOuterRadiusUnits=m  ExtGeomFileType=STL  ExtGeomFileName=hip_shaft.stl  ExtGeomFileUnits=m  RevolutionCrossSection=[1 1; 1 -1; 2 -1; 2 1]  RevolutionCrossSectionUnits=m  RevolutionExtent=Full  RevolutionAngle=180  RevolutionAngleUnits=deg  BlockFunction=simmechanics.library.body_elements.solid
  CS1 : PMIOPort  Port=1  Side=Left
  CS2 : PMIOPort  Port=2  Side=Right
  connections:
  CS2/RConn1 -- Rotate back 180 degrees/RConn1
  CS1 to CS2/LConn1 -- Frame Data/LConn1 -- Rotate 180 degrees/RConn1 -- Solid/RConn1
  Rotate 180 degrees/LConn1 -- CS1/RConn1
  Rotate back 180 degrees/LConn1 -- CS1 to CS2/RConn1

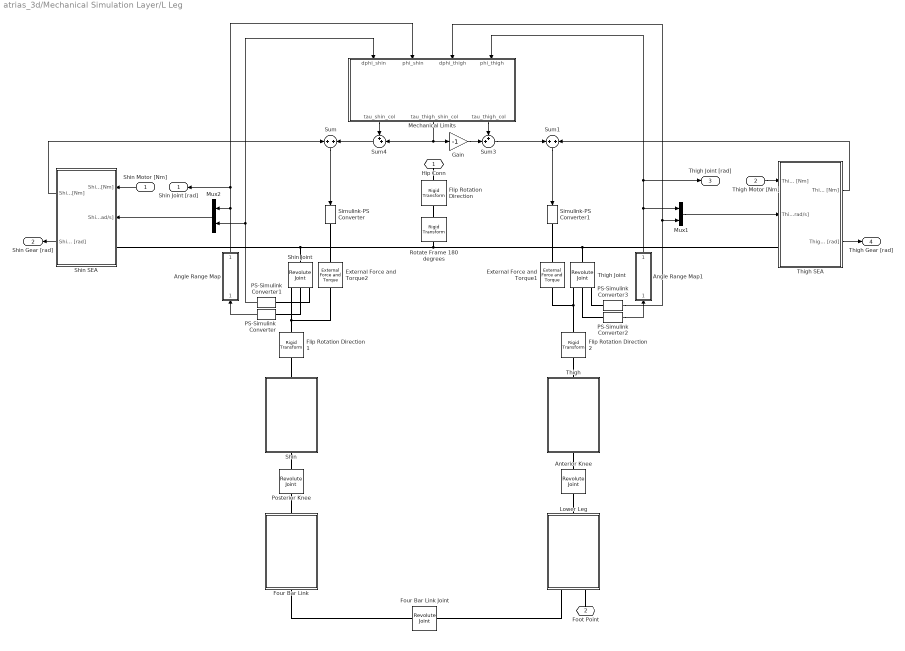
== system atrias_3d/Mechanical Simulation Layer/L Leg ==
  Shin Motor [Nm] : Inport
  "Thigh Motor [Nm]  " : Inport  Port=2
  Angle Range Map : Subsystem
  Angle Range Map1 : Subsystem
  Anterior Knee : sm_lib/Joints/Revolute Joint  SenseConstraintForce=off  SenseConstraintForceX=off  SenseConstraintForceY=off  SenseConstraintForceZ=off  SenseConstraintTorque=off  SenseConstraintTorqueX=off  SenseConstraintTorqueY=off  SenseConstraintTorqueZ=off  SenseTotalForce=off  SenseTotalForceX=off  SenseTotalForceY=off  SenseTotalForceZ=off  SenseTotalTorque=off  SenseTotalTorqueX=off  SenseTotalTorqueY=off  SenseTotalTorqueZ=off  CompositeWrenchDir=FollowerOnBase  CompositeWrenchFrame=BaseFrame  EquilibriumPosition=0  EquilibriumPositionUnits=deg  SpringStiffness=0  SpringStiffnessUnits=N*m/deg  DampingCoefficient=0  DampingCoefficientUnits=N*m/(deg/s)  TorqueActuationMode=NoTorque  MotionActuationMode=ComputedMotion  SensePosition=off  SenseVelocity=off  SenseAcceleration=off  SenseTorqueForce=off  PositionTargetValue=30  PositionTargetValueUnits=deg  PositionTargetSpecify=off  PositionTargetPriority=Low  VelocityTargetValue=0  VelocityTargetValueUnits=deg/s  VelocityTargetSpecify=off  VelocityTargetPriority=High  BlockFunction=simmechanics.library.joints.revolute_joint
  External Force and Torque1 : sm_lib/Forces and Torques/External Force and Torque  ForceResolutionFrame=AttachedFrame  EnableForceX=off  EnableForceY=off  EnableForceZ=off  EnableForce=off  TorqueResolutionFrame=AttachedFrame  EnableTorqueX=off  EnableTorqueY=off  EnableTorqueZ=on  EnableTorque=off  BlockFunction=simmechanics.library.forces_torques.external_force_torque
  External Force and Torque2 : sm_lib/Forces and Torques/External Force and Torque  ForceResolutionFrame=AttachedFrame  EnableForceX=off  EnableForceY=off  EnableForceZ=off  EnableForce=off  TorqueResolutionFrame=AttachedFrame  EnableTorqueX=off  EnableTorqueY=off  EnableTorqueZ=on  EnableTorque=off  BlockFunction=simmechanics.library.forces_torques.external_force_torque
  Flip Rotation Direction : sm_lib/Frames and Transforms/Rigid Transform  TranslationMethod=None  TranslationLengthUnit=m  TranslationStandardAxis=+Z  TranslationStandardOffset=0  TranslationCartesianOffset=[0 0 0]  TranslationROffset=0  TranslationROffsetUnits=m  TranslationZOffset=0  TranslationZOffsetUnits=m  TranslationThetaOffset=0  TranslationThetaOffsetUnits=deg  RotationMethod=AlignedAxes  RotationAngleUnits=deg  RotationStandardAxis=-Z  RotationAngle=180  RotationArbitraryAxis=[0 0 1]  FollAlignAxisA=-Z  BaseAlignAxisA=+Z  FollAlignAxisB=+Y  BaseAlignAxisB=+Y  RotationMatrix=[1 0 0; 0 1 0; 0 0 1]  BlockFunction=simmechanics.library.frames_transforms.rigid_transform
  Flip Rotation Direction 1 : sm_lib/Frames and Transforms/Rigid Transform  TranslationMethod=None  TranslationLengthUnit=m  TranslationStandardAxis=+Z  TranslationStandardOffset=0  TranslationCartesianOffset=[0 0 0]  TranslationROffset=0  TranslationROffsetUnits=m  TranslationZOffset=0  TranslationZOffsetUnits=m  TranslationThetaOffset=0  TranslationThetaOffsetUnits=deg  RotationMethod=AlignedAxes  RotationAngleUnits=deg  RotationStandardAxis=-Z  RotationAngle=180  RotationArbitraryAxis=[0 0 1]  FollAlignAxisA=-Z  BaseAlignAxisA=+Z  FollAlignAxisB=+Y  BaseAlignAxisB=+Y  RotationMatrix=[1 0 0; 0 1 0; 0 0 1]  BlockFunction=simmechanics.library.frames_transforms.rigid_transform
  Flip Rotation Direction 2 : sm_lib/Frames and Transforms/Rigid Transform  TranslationMethod=None  TranslationLengthUnit=m  TranslationStandardAxis=+Z  TranslationStandardOffset=0  TranslationCartesianOffset=[0 0 0]  TranslationROffset=0  TranslationROffsetUnits=m  TranslationZOffset=0  TranslationZOffsetUnits=m  TranslationThetaOffset=0  TranslationThetaOffsetUnits=deg  RotationMethod=AlignedAxes  RotationAngleUnits=deg  RotationStandardAxis=-Z  RotationAngle=180  RotationArbitraryAxis=[0 0 1]  FollAlignAxisA=-Z  BaseAlignAxisA=+Z  FollAlignAxisB=+Y  BaseAlignAxisB=+Y  RotationMatrix=[1 0 0; 0 1 0; 0 0 1]  BlockFunction=simmechanics.library.frames_transforms.rigid_transform
  Four Bar Link : Subsystem
      mask Display: image('four_bar_link.jpg');
  Four Bar Link Joint : sm_lib/Joints/Revolute Joint  SenseConstraintForce=off  SenseConstraintForceX=off  SenseConstraintForceY=off  SenseConstraintForceZ=off  SenseConstraintTorque=off  SenseConstraintTorqueX=off  SenseConstraintTorqueY=off  SenseConstraintTorqueZ=off  SenseTotalForce=off  SenseTotalForceX=off  SenseTotalForceY=off  SenseTotalForceZ=off  SenseTotalTorque=off  SenseTotalTorqueX=off  SenseTotalTorqueY=off  SenseTotalTorqueZ=off  CompositeWrenchDir=FollowerOnBase  CompositeWrenchFrame=BaseFrame  EquilibriumPosition=0  EquilibriumPositionUnits=deg  SpringStiffness=0  SpringStiffnessUnits=N*m/deg  DampingCoefficient=0  DampingCoefficientUnits=N*m/(deg/s)  TorqueActuationMode=NoTorque  MotionActuationMode=ComputedMotion  SensePosition=off  SenseVelocity=off  SenseAcceleration=off  SenseTorqueForce=off  PositionTargetValue=30  PositionTargetValueUnits=deg  PositionTargetSpecify=off  PositionTargetPriority=Low  VelocityTargetValue=0  VelocityTargetValueUnits=deg/s  VelocityTargetSpecify=off  VelocityTargetPriority=High  BlockFunction=simmechanics.library.joints.revolute_joint
  Gain : Gain  Gain=-1
  Lower Leg : Subsystem
      mask Display: image('lower_leg.jpg');
  Mechanical Limits : Subsystem
      settings: MinAlgLoopOccurrences=on
  Mux1 : Mux  Inputs=2
  Mux2 : Mux  Inputs=2
  PS-Simulink Converter{,1..3} (4 alike) : nesl_utility/PS-Simulink Converter  PhysicalDomain=network_engine_domain  SubClassName=ps_output  LeftPortType=input  RightPortType=output  PseudoPeriodic=off  Frequencies=[]  Unit=1  AffineConversion=off
  Posterior Knee : sm_lib/Joints/Revolute Joint  SenseConstraintForce=off  SenseConstraintForceX=off  SenseConstraintForceY=off  SenseConstraintForceZ=off  SenseConstraintTorque=off  SenseConstraintTorqueX=off  SenseConstraintTorqueY=off  SenseConstraintTorqueZ=off  SenseTotalForce=off  SenseTotalForceX=off  SenseTotalForceY=off  SenseTotalForceZ=off  SenseTotalTorque=off  SenseTotalTorqueX=off  SenseTotalTorqueY=off  SenseTotalTorqueZ=off  CompositeWrenchDir=FollowerOnBase  CompositeWrenchFrame=BaseFrame  EquilibriumPosition=0  EquilibriumPositionUnits=deg  SpringStiffness=0  SpringStiffnessUnits=N*m/deg  DampingCoefficient=0  DampingCoefficientUnits=N*m/(deg/s)  TorqueActuationMode=NoTorque  MotionActuationMode=ComputedMotion  SensePosition=off  SenseVelocity=off  SenseAcceleration=off  SenseTorqueForce=off  PositionTargetValue=30  PositionTargetValueUnits=deg  PositionTargetSpecify=off  PositionTargetPriority=Low  VelocityTargetValue=0  VelocityTargetValueUnits=deg/s  VelocityTargetSpecify=off  VelocityTargetPriority=High  BlockFunction=simmechanics.library.joints.revolute_joint
  Rotate Frame 180 degrees : sm_lib/Frames and Transforms/Rigid Transform  TranslationMethod=None  TranslationLengthUnit=m  TranslationStandardAxis=+Z  TranslationStandardOffset=0  TranslationCartesianOffset=[0 0 0]  TranslationROffset=0  TranslationROffsetUnits=m  TranslationZOffset=0  TranslationZOffsetUnits=m  TranslationThetaOffset=0  TranslationThetaOffsetUnits=deg  RotationMethod=StandardAxis  RotationAngleUnits=deg  RotationStandardAxis=+Z  RotationAngle=180  RotationArbitraryAxis=[0 0 1]  FollAlignAxisA=-Z  BaseAlignAxisA=+Z  FollAlignAxisB=+Y  BaseAlignAxisB=+Y  RotationMatrix=[1 0 0; 0 1 0; 0 0 1]  BlockFunction=simmechanics.library.frames_transforms.rigid_transform
  Shin : Subsystem
      mask Display: image('shin.jpg');
  Shin Joint : sm_lib/Joints/Revolute Joint  SenseConstraintForce=off  SenseConstraintForceX=off  SenseConstraintForceY=off  SenseConstraintForceZ=off  SenseConstraintTorque=off  SenseConstraintTorqueX=off  SenseConstraintTorqueY=off  SenseConstraintTorqueZ=off  SenseTotalForce=off  SenseTotalForceX=off  SenseTotalForceY=off  SenseTotalForceZ=off  SenseTotalTorque=off  SenseTotalTorqueX=off  SenseTotalTorqueY=off  SenseTotalTorqueZ=off  CompositeWrenchDir=FollowerOnBase  CompositeWrenchFrame=BaseFrame  EquilibriumPosition=0  EquilibriumPositionUnits=deg  SpringStiffness=0  SpringStiffnessUnits=N*m/deg  DampingCoefficient=0  DampingCoefficientUnits=N*m/(deg/s)  TorqueActuationMode=NoTorque  MotionActuationMode=ComputedMotion  SensePosition=on  SenseVelocity=on  SenseAcceleration=off  SenseTorqueForce=off  PositionTargetValue=shin_initial_l  PositionTargetValueUnits=rad  PositionTargetSpecify=on  PositionTargetPriority=High  VelocityTargetValue=0  VelocityTargetValueUnits=deg/s  VelocityTargetSpecify=off  VelocityTargetPriority=High  BlockFunction=simmechanics.library.joints.revolute_joint
  Shin SEA : Subsystem
      mask Display: image('shin_sea.jpg')
  Simulink-PS Converter : nesl_utility/Simulink-PS Converter  PhysicalDomain=network_engine_domain  SubClassName=ps_input  LeftPortType=input  RightPortType=output  PseudoPeriodic=off  Frequencies=[]  NoiseDistribution=none  NoiseParameters=[]  Unit=1  AffineConversion=off  InputFiltering=off  SimscapeFilterOrder=1  InputFilterTimeConstant=0.001  UdotUserProvided=1
  Simulink-PS Converter1 : nesl_utility/Simulink-PS Converter  PhysicalDomain=network_engine_domain  SubClassName=ps_input  LeftPortType=input  RightPortType=output  PseudoPeriodic=off  Frequencies=[]  NoiseDistribution=none  NoiseParameters=[]  Unit=1  AffineConversion=off  InputFiltering=off  SimscapeFilterOrder=1  InputFilterTimeConstant=0.001  UdotUserProvided=1
  Sum : Sum  Inputs=+|+
  Sum1 : Sum  Inputs=+|+
  Sum3 : Sum  Inputs=++|
  Sum4 : Sum  Inputs=++|
  Thigh : Subsystem
      mask Display: image('thigh.jpg');
  Thigh Joint : sm_lib/Joints/Revolute Joint  SenseConstraintForce=off  SenseConstraintForceX=off  SenseConstraintForceY=off  SenseConstraintForceZ=off  SenseConstraintTorque=off  SenseConstraintTorqueX=off  SenseConstraintTorqueY=off  SenseConstraintTorqueZ=off  SenseTotalForce=off  SenseTotalForceX=off  SenseTotalForceY=off  SenseTotalForceZ=off  SenseTotalTorque=off  SenseTotalTorqueX=off  SenseTotalTorqueY=off  SenseTotalTorqueZ=off  CompositeWrenchDir=FollowerOnBase  CompositeWrenchFrame=BaseFrame  EquilibriumPosition=0  EquilibriumPositionUnits=deg  SpringStiffness=0  SpringStiffnessUnits=N*m/deg  DampingCoefficient=0  DampingCoefficientUnits=N*m/(deg/s)  TorqueActuationMode=NoTorque  MotionActuationMode=ComputedMotion  SensePosition=on  SenseVelocity=on  SenseAcceleration=off  SenseTorqueForce=off  PositionTargetValue=thigh_initial_l  PositionTargetValueUnits=rad  PositionTargetSpecify=on  PositionTargetPriority=High  VelocityTargetValue=0  VelocityTargetValueUnits=deg/s  VelocityTargetSpecify=off  VelocityTargetPriority=High  BlockFunction=simmechanics.library.joints.revolute_joint
  Thigh SEA : Subsystem
      mask Display: image('thigh_sea.jpg')
  Hip Conn : PMIOPort  Port=1  Side=Left
  Foot Point : PMIOPort  Port=2  Side=Right
  Shin Joint [rad] : Outport
  Shin Gear [rad] : Outport  Port=2
  Thigh Joint [rad] : Outport  Port=3
  Thigh Gear [rad] : Outport  Port=4
  wires:
  Angle Range Map1/1("[0,2*pi]") -> Mux1/1, Thigh Joint [rad]/1, Mechanical Limits/4(phi_thigh)
  Mux2/1 -> Shin SEA/2(Shin Joint [rad rad/s])
  Sum/1 -> Simulink-PS Converter/1
  Sum4/1 -> Sum/2
  Sum3/1 -> Sum1/1
  Mechanical Limits/1(tau_shin_col) -> Sum4/1
  Mechanical Limits/3(tau_thigh_col) -> Sum3/1
  Gain/1 -> Sum3/2
  Shin SEA/2(Shin Gear [rad]) -> Shin Gear [rad]/1
  Thigh SEA/2(Thigh Gear [rad]) -> Thigh Gear [rad]/1
  Mux1/1 -> Thigh SEA/2(Thigh Joint [rad rad/s])
  PS-Simulink Converter1/1 -> Mux2/2, Mechanical Limits/1(dphi_shin)
  Mechanical Limits/2(tau_thigh_shin_col) -> Sum4/2, Gain/1
  PS-Simulink Converter3/1 -> Mux1/2, Mechanical Limits/3(dphi_thigh)
  Thigh SEA/1(Thigh Joint Torque [Nm]) -> Sum1/2
  Sum1/1 -> Simulink-PS Converter1/1
  Shin SEA/1(Shin Joint Torque [Nm]) -> Sum/1
  PS-Simulink Converter2/1 -> Angle Range Map1/1("[-pi, pi]")
  Angle Range Map/1("[0,2*pi]") -> Mux2/1, Shin Joint [rad]/1, Mechanical Limits/2(phi_shin)
  PS-Simulink Converter/1 -> Angle Range Map/1("[-pi, pi]")
  Shin Motor [Nm]/1 -> Shin SEA/1(Shin Gear Torque [Nm])
  "Thigh Motor [Nm]  "/1 -> Thigh SEA/1(Thigh Gear Torque [Nm])
  connections:
  Simulink-PS Converter1/RConn1 -- External Force and Torque1/LConn1
  PS-Simulink Converter2/LConn1 -- Thigh Joint/RConn2
  PS-Simulink Converter3/LConn1 -- Thigh Joint/RConn3
  Flip Rotation Direction/RConn1 -- Rotate Frame 180 degrees/LConn1
  Flip Rotation Direction 2/RConn1 -- Thigh/LConn1
  Flip Rotation Direction 1/RConn1 -- Shin/LConn1
  Flip Rotation Direction/LConn1 -- Hip Conn/RConn1
  Thigh Joint/LConn1 -- Thigh SEA/LConn1 -- Shin Joint/LConn1 -- Shin SEA/LConn1 -- Rotate Frame 180 degrees/RConn1
  PS-Simulink Converter1/LConn1 -- Shin Joint/RConn3
  PS-Simulink Converter/LConn1 -- Shin Joint/RConn2
  Simulink-PS Converter/RConn1 -- External Force and Torque2/LConn1
  Posterior Knee/LConn1 -- Shin/RConn1
  External Force and Torque1/RConn1 -- Flip Rotation Direction 2/LConn1 -- Thigh Joint/RConn1
  External Force and Torque2/RConn1 -- Flip Rotation Direction 1/LConn1 -- Shin Joint/RConn1
  Anterior Knee/LConn1 -- Thigh/RConn1
  Lower Leg/LConn1 -- Anterior Knee/RConn1
  Lower Leg/RConn2 -- Foot Point/RConn1
  Four Bar Link Joint/RConn1 -- Four Bar Link/RConn1
  Posterior Knee/RConn1 -- Four Bar Link/LConn1
  Four Bar Link Joint/LConn1 -- Lower Leg/RConn1
